simulink model "pendulum_animation"  (Simulink 8.3)
settings: Solver=ode45  StartTime=0.0  StopTime=10000  RelTol=1e-3
undefined symbols (not defined in the file or in its folder): drawPendulum
libraries: simulink x3
settings Model: Creator=beard  LastModifiedBy=jhl48
settings OptimizationCC: ExpressionDepthLimit=2147483647  InitFltsAndDblsToZero=on
settings DebuggingCC: FcnCallInpInsideContextMsg=UseLocalSettings

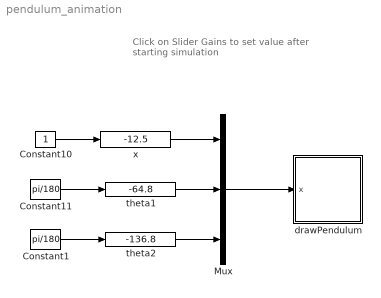
== system pendulum_animation ==
  note: Click on Slider Gains to set value
      | after starting simulation
  Constant1 : Constant  Value=pi/180
  Constant10 : Constant
  Constant11 : Constant  Value=pi/180
  Mux : Mux  Inputs=3
  drawPendulum : Subsystem
      mask init:
      | % drawing parameters
      | L = 1;
      | gap = 0.01;
      | width = 1.0;
      | height = 0.1;
      mask Display: image(imread('tv.jpg'))
  theta1 : simulink/Math Operations/Slider Gain  low=-180  gain=-64.8  high=180
  theta2 : simulink/Math Operations/Slider Gain  low=-180  gain=-136.8  high=180
  x : simulink/Math Operations/Slider Gain  low=-50  gain=-12.5  high=0
  wires:
  x/1 -> Mux/1
  Constant10/1 -> x/1
  theta1/1 -> Mux/2
  Constant11/1 -> theta1/1
  Mux/1 -> drawPendulum/1(x)
  Constant1/1 -> theta2/1
  theta2/1 -> Mux/3

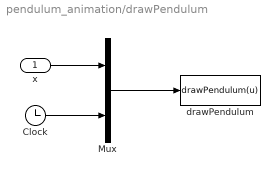
== system pendulum_animation/drawPendulum ==
  x : Inport
  Clock : Clock
  Mux : Mux  Inputs=2
  drawPendulum : MATLABFcn  MATLABFcn=drawPendulum(u)  OutputDimensions=0  SampleTime=0.1
  wires:
  Mux/1 -> drawPendulum/1
  x/1 -> Mux/1
  Clock/1 -> Mux/2
